simulink model "hw3b_sim"  (Simulink 9.2)
settings: Solver=ode5  StartTime=0.0  StopTime=10  FixedStep=0.001  RelTol=1e-3
values from neighbouring files (symbols this model uses):
  a = 1.14    [hw3b.m]
  b = L-a    (= 1.4)    [hw3b.m]
  Cf = 44000*2    (= 88000)    [hw3b.m]
  Cr = 47000*2    (= 94000)    [hw3b.m]
  Iz = 2420.0    (= 2420)    [hw3b.m]
  KD = 0.105    [hw3b.m]
  KP = 0.610    (= 0.61)    [hw3b.m]
  m = 1500    [hw3b.m]
  s = 0:0.1:600    [road_shape.m]
  TT = 0.04    [hw3b.m]
  x0 = cumtrapz(s, 1./sqrt(1+grad.^2))    [road_shape.m]
  y0 = cumtrapz(s, grad./sqrt(1+grad.^2))    [road_shape.m]
undefined symbols (not defined in the file or in its folder): DiscIntNeverNeededParam
libraries: simulink x2
settings Model: Creator=Changsun Ahn  LastModifiedBy=Changsun Ahn
settings DataIOCC: SignalLoggingName=sigsOut
settings OptimizationCC: ExpressionDepthLimit=2147483647
settings DebuggingCC: SaveWithParameterizedLinksMsg=none  SignalResolutionControl=TryResolveAllWithWarning  MultiTaskDSMMsg=warning  MultiTaskCondExecSysMsg=none  FcnCallInpInsideContextMsg=error
settings HardwareCC: TargetBitPerPointer=64  TargetBitPerSizeT=64  TargetBitPerPtrDiffT=64  TargetLongLongMode=on  TargetIntDivRoundTo=Zero  TargetEndianess=LittleEndian  TargetWordSize=64  TargetHWDeviceType=MATLAB Host  ProdEqTarget=off

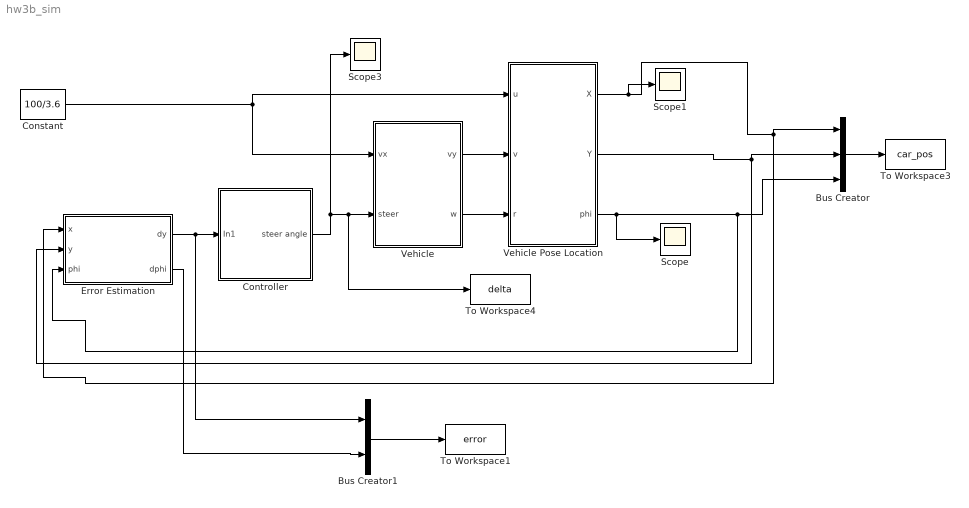
== system hw3b_sim ==
  Bus Creator : BusCreator  Inputs=3
  Bus Creator1 : BusCreator  Inputs=2
  Constant : Constant  Value=100/3.6
  Controller : Subsystem
  Error Estimation : Subsystem
  Scope : Scope
  Scope1 : Scope
  Scope3 : Scope
  To Workspace1 : ToWorkspace  VariableName=error  SaveFormat=Timeseries  SampleTime=-1
  To Workspace3 : ToWorkspace  VariableName=car_pos  SaveFormat=Timeseries  SampleTime=-1
  To Workspace4 : ToWorkspace  VariableName=delta  SaveFormat=Timeseries  SampleTime=-1
  Vehicle : Subsystem
  Vehicle Pose Location : Subsystem
  wires:
  Vehicle/1(vy) -> Vehicle Pose Location/2(v)
  Vehicle/2(w) -> Vehicle Pose Location/3(r)
  Vehicle Pose Location/3(phi) -> Error Estimation/3(phi), Bus Creator/3, Scope/1
  Constant/1 -> Vehicle Pose Location/1(u), Vehicle/1(vx)
  Vehicle Pose Location/1(X) -> Scope1/1, Error Estimation/1(x), Bus Creator/1
  Controller/1(steer angle) -> Scope3/1, To Workspace4/1, Vehicle/2(steer)
  Vehicle Pose Location/2(Y) -> Error Estimation/2(y), Bus Creator/2
  Bus Creator/1 -> To Workspace3/1
  Error Estimation/1(dy) -> Bus Creator1/1, Controller/1(In1)
  Error Estimation/2(dphi) -> Bus Creator1/2
  Bus Creator1/1 -> To Workspace1/1

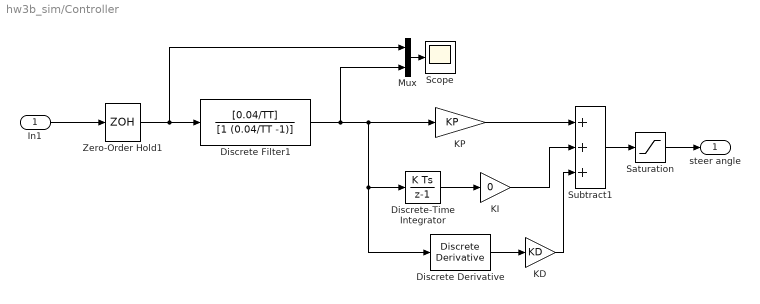
== system hw3b_sim/Controller ==
  In1 : Inport
  Discrete Derivative : simulink/Discrete/Discrete Derivative  gainval=1.0  ICPrevScaledInput=0.0  OutMin=[]  OutMax=[]  OutDataType=fixdt(1, 16)  OutScaling=2^-10  DoSatur=off
  Discrete Filter1 : DiscreteFilter  Numerator=[0.04/TT]  Denominator=[1 (0.04/TT -1)]
  Discrete-Time Integrator : DiscreteIntegrator  SampleTime=-1  ICPrevOutput=DiscIntNeverNeededParam  ICPrevScaledInput=DiscIntNeverNeededParam
  KD : Gain  Gain=KD
  KI : Gain  Gain=0
  KP : Gain  Gain=KP
  Mux : Mux  Inputs=2
  Saturation : Saturate  UpperLimit=30*pi/180  LowerLimit=-30*pi/180
  Scope : Scope
  Subtract1 : Sum  Inputs=+++
  Zero-Order Hold1 : ZeroOrderHold  SampleTime=0.04
  steer angle : Outport
  wires:
  Saturation/1 -> steer angle/1
  Discrete-Time Integrator/1 -> KI/1
  KD/1 -> Subtract1/3
  Discrete Derivative/1 -> KD/1
  KP/1 -> Subtract1/1
  KI/1 -> Subtract1/2
  In1/1 -> Zero-Order Hold1/1
  Mux/1 -> Scope/1
  Discrete Filter1/1 -> Mux/2, Discrete Derivative/1, Discrete-Time Integrator/1, KP/1
  Zero-Order Hold1/1 -> Mux/1, Discrete Filter1/1
  Subtract1/1 -> Saturation/1

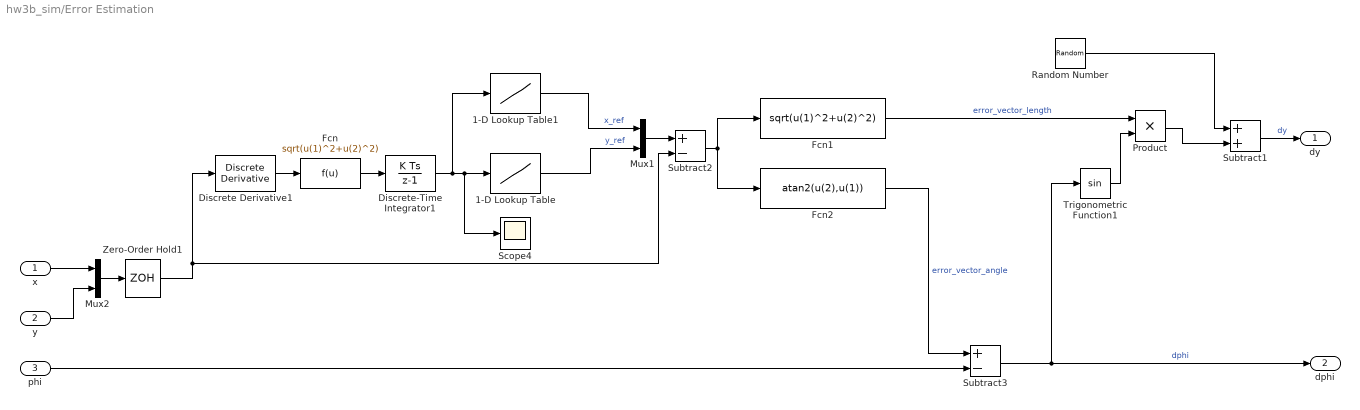
== system hw3b_sim/Error Estimation ==
  x : Inport
  y : Inport  Port=2
  phi : Inport  Port=3
  1-D Lookup Table : Lookup_n-D  NumberOfTableDimensions=1  BreakpointsForDimension1=s  Table=y0  InternalRulePriority=Speed  RndMeth=Simplest  InputSameDT=on
  1-D Lookup Table1 : Lookup_n-D  NumberOfTableDimensions=1  BreakpointsForDimension1=s  Table=x0  InternalRulePriority=Speed  RndMeth=Simplest  InputSameDT=on
  Discrete Derivative1 : simulink/Discrete/Discrete Derivative  gainval=1.0  ICPrevScaledInput=0.0  OutMin=[]  OutMax=[]  OutDataType=fixdt(1, 16)  OutScaling=2^-10  DoSatur=off
  Discrete-Time Integrator1 : DiscreteIntegrator  SampleTime=-1  ICPrevOutput=DiscIntNeverNeededParam  ICPrevScaledInput=DiscIntNeverNeededParam
  Fcn : Fcn  Expr=sqrt(u(1)^2+u(2)^2)
  Fcn1 : Fcn  Expr=sqrt(u(1)^2+u(2)^2)
  Fcn2 : Fcn  Expr=atan2(u(2),u(1))
  Mux1 : Mux  Inputs=2
  Mux2 : Mux  Inputs=2
  Product : Product
  Random Number : RandomNumber  Variance=0.002*0  SampleTime=0.04
  Scope4 : Scope
  Subtract1 : Sum
  Subtract2 : Sum  Inputs=+-
  Subtract3 : Sum  Inputs=+-
  Trigonometric Function1 : Trigonometry
  Zero-Order Hold1 : ZeroOrderHold  SampleTime=0.04
  dy : Outport
  dphi : Outport  Port=2
  wires:
  Subtract3/1 -> Trigonometric Function1/1, dphi/1  "dphi"
  Discrete-Time Integrator1/1 -> 1-D Lookup Table/1, Scope4/1, 1-D Lookup Table1/1
  phi/1 -> Subtract3/2
  Subtract2/1 -> Fcn2/1, Fcn1/1
  x/1 -> Mux2/1
  Trigonometric Function1/1 -> Product/2
  Fcn1/1 -> Product/1  "error_vector_length"
  1-D Lookup Table1/1 -> Mux1/1  "x_ref"
  Mux2/1 -> Zero-Order Hold1/1
  Fcn2/1 -> Subtract3/1  "error_vector_angle"
  Mux1/1 -> Subtract2/1
  Fcn/1 -> Discrete-Time Integrator1/1
  1-D Lookup Table/1 -> Mux1/2  "y_ref"
  Subtract1/1 -> dy/1  "dy"
  Random Number/1 -> Subtract1/1
  Product/1 -> Subtract1/2
  Discrete Derivative1/1 -> Fcn/1
  Zero-Order Hold1/1 -> Subtract2/2, Discrete Derivative1/1
  y/1 -> Mux2/2

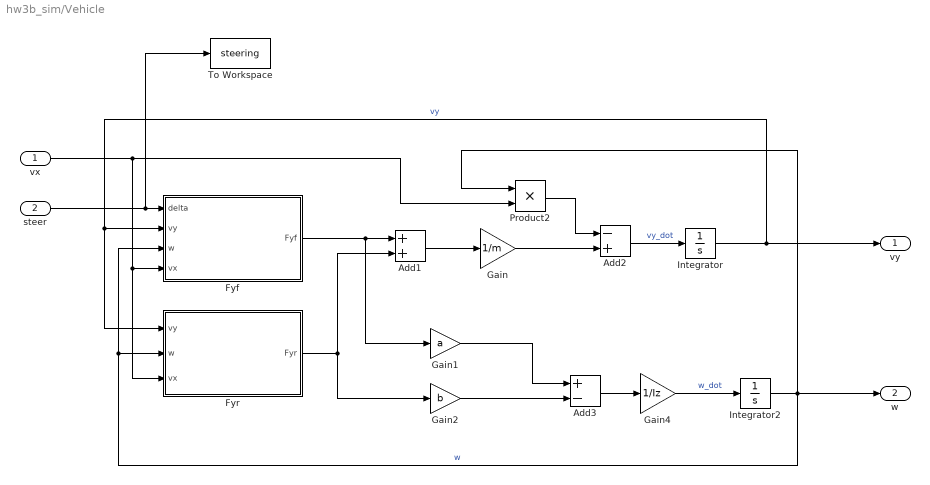
== system hw3b_sim/Vehicle ==
  vx : Inport
  steer : Inport  Port=2
  Add1 : Sum
  Add2 : Sum  Inputs=-+
  Add3 : Sum  Inputs=+-
  Fyf : Subsystem
  Fyr : Subsystem
  Gain : Gain  Gain=1/m
  Gain1 : Gain  Gain=a
  Gain2 : Gain  Gain=b
  Gain4 : Gain  Gain=1/Iz
  Integrator : Integrator
  Integrator2 : Integrator
  Product2 : Product  RndMeth=Zero
  To Workspace : ToWorkspace  VariableName=steering  SaveFormat=Timeseries  SampleTime=-1
  vy : Outport
  w : Outport  Port=2
  wires:
  Add1/1 -> Gain/1
  Gain/1 -> Add2/2
  vx/1 -> Fyr/3(vx), Fyf/4(vx), Product2/2
  Product2/1 -> Add2/1
  Add2/1 -> Integrator/1  "vy_dot"
  Fyf/1(Fyf) -> Gain1/1, Add1/1
  Fyr/1(Fyr) -> Gain2/1, Add1/2
  Integrator/1 -> vy/1, Fyf/2(vy), Fyr/1(vy)  "vy"
  Gain1/1 -> Add3/1
  Gain2/1 -> Add3/2
  Add3/1 -> Gain4/1
  Gain4/1 -> Integrator2/1  "w_dot"
  Integrator2/1 -> w/1, Product2/1, Fyf/3(w), Fyr/2(w)  "w"
  steer/1 -> To Workspace/1, Fyf/1(delta)

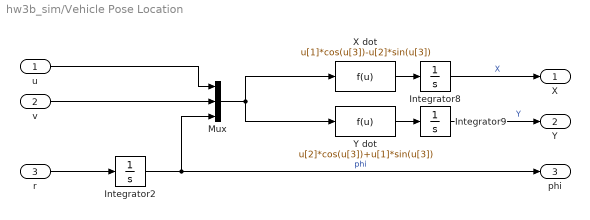
== system hw3b_sim/Vehicle Pose Location ==
  u : Inport
  v : Inport  Port=2
  r : Inport  Port=3
  Integrator2 : Integrator
  Integrator8 : Integrator
  Integrator9 : Integrator
  Mux : Mux  Inputs=3
  X dot : Fcn  Expr=u[1]*cos(u[3])-u[2]*sin(u[3])
  Y dot : Fcn  Expr=u[2]*cos(u[3])+u[1]*sin(u[3])  SampleTime=0
  X : Outport
  Y : Outport  Port=2
  phi : Outport  Port=3
  wires:
  r/1 -> Integrator2/1
  Integrator2/1 -> phi/1, Mux/3  "phi"
  Mux/1 -> Y dot/1, X dot/1
  Y dot/1 -> Integrator9/1
  X dot/1 -> Integrator8/1
  Integrator9/1 -> Y/1  "Y"
  Integrator8/1 -> X/1  "X"
  v/1 -> Mux/2
  u/1 -> Mux/1

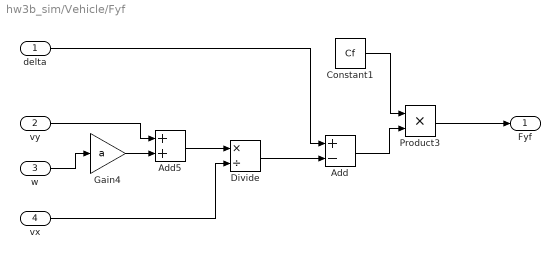
== system hw3b_sim/Vehicle/Fyf ==
  delta : Inport
  vy : Inport  Port=2
  w : Inport  Port=3
  vx : Inport  Port=4
  Add : Sum  Inputs=+-
  Add5 : Sum
  Constant1 : Constant  Value=Cf
  Divide : Product  Inputs=*/
  Gain4 : Gain  Gain=a
  Product3 : Product  RndMeth=Zero
  Fyf : Outport
  wires:
  w/1 -> Gain4/1
  vy/1 -> Add5/1
  Add5/1 -> Divide/1
  Gain4/1 -> Add5/2
  vx/1 -> Divide/2
  Constant1/1 -> Product3/1
  Add/1 -> Product3/2
  Divide/1 -> Add/2
  delta/1 -> Add/1
  Product3/1 -> Fyf/1

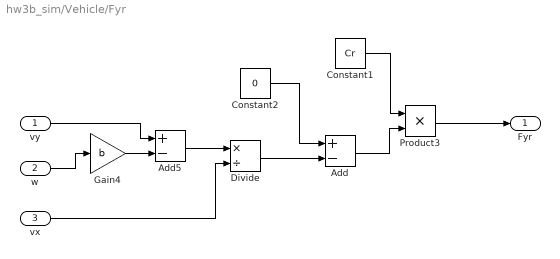
== system hw3b_sim/Vehicle/Fyr ==
  vy : Inport
  w : Inport  Port=2
  vx : Inport  Port=3
  Add : Sum  Inputs=+-
  Add5 : Sum  Inputs=+-
  Constant1 : Constant  Value=Cr
  Constant2 : Constant  Value=0
  Divide : Product  Inputs=*/
  Gain4 : Gain  Gain=b
  Product3 : Product  RndMeth=Zero
  Fyr : Outport
  wires:
  w/1 -> Gain4/1
  vy/1 -> Add5/1
  Add5/1 -> Divide/1
  Gain4/1 -> Add5/2
  vx/1 -> Divide/2
  Constant1/1 -> Product3/1
  Add/1 -> Product3/2
  Divide/1 -> Add/2
  Product3/1 -> Fyr/1
  Constant2/1 -> Add/1
